simulink model "simulacion_validacion"  (R2022b)
settings: Solver=VariableStepAuto  StartTime=0.0  StopTime=50  RelTol=1e-3
values from neighbouring files (symbols this model uses):
  beta = gamma*2*I    (= 0.0001265)    [parametros.m]
  db = 4.2/100    (= 0.042)    [parametros.m]
  dc = 5/100    (= 0.05)    [parametros.m]
  dm = 13.1/100    (= 0.131)    [parametros.m]
  g = 9.81    [parametros.m]
  I = 1.1e-4    (= 0.00011)    [parametros.m]
  K = 0.001    [parametros.m]
  mb = 7.38/1000    (= 0.00738)    [parametros.m]
  mc = 2.07/1000    (= 0.00207)    [parametros.m]
  mm = (3.2+1.28)/1000    (= 0.00448)    [parametros.m]
settings Model: Creator=TAURET  LastModifiedBy=danie
settings DataIOCC: Refine=100
settings ModelReferenceCC: EnableRefExpFcnMdlSchedulingChecks=on

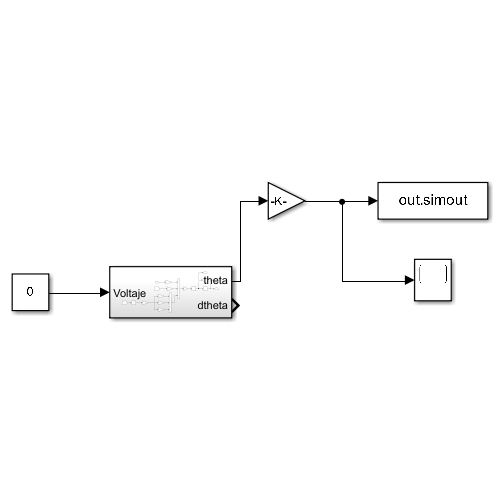
[thumbnail: Simulink's stored preview of the top-level diagram]
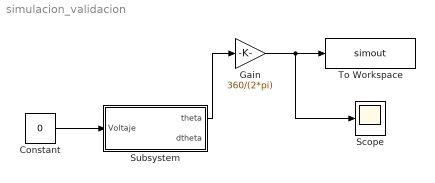
== system simulacion_validacion ==
  Constant : Constant  Value=0
  Gain : Gain  Gain=360/(2*pi)
  Scope : Scope
  Subsystem : Subsystem
  To Workspace : ToWorkspace  VariableName=simout  SaveFormat=Timeseries  SampleTime=-1
  wires:
  Subsystem/1(theta) -> Gain/1
  Gain/1 -> To Workspace/1, Scope/1
  Constant/1 -> Subsystem/1(Voltaje)

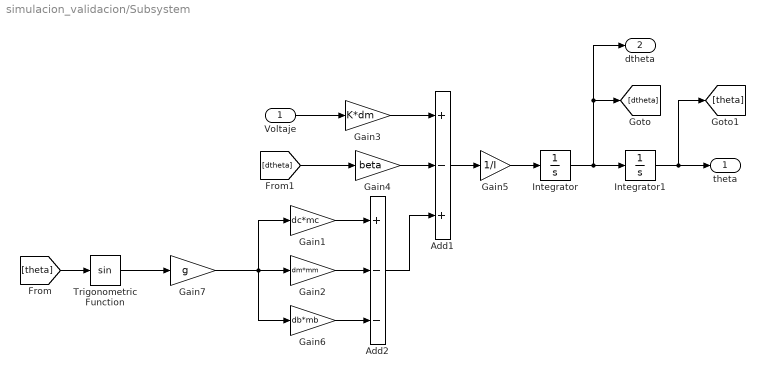
== system simulacion_validacion/Subsystem ==
  Voltaje : Inport
  Add1 : Sum  Inputs=+-+
  Add2 : Sum  Inputs=+--
  Gain1 : Gain  Gain=dc*mc
  Gain2 : Gain  Gain=dm*mm
  Gain3 : Gain  Gain=K*dm
  Gain4 : Gain  Gain=beta
  Gain5 : Gain  Gain=1/I
  Gain6 : Gain  Gain=db*mb
  Gain7 : Gain  Gain=g
  Integrator : Integrator
  Integrator1 : Integrator  InitialCondition=1.57
  Trigonometric Function : Trigonometry
  theta : Outport
  dtheta : Outport  Port=2
  wires:
  Gain4/1 -> Add1/2
  Gain5/1 -> Integrator/1
  Add1/1 -> Gain5/1
  [dtheta] -> Gain4/1
  [theta] -> Trigonometric Function/1
  Integrator/1 -> dtheta/1, [dtheta], Integrator1/1
  Integrator1/1 -> [theta], theta/1
  Voltaje/1 -> Gain3/1
  Gain1/1 -> Add2/1
  Gain2/1 -> Add2/2
  Gain6/1 -> Add2/3
  Add2/1 -> Add1/3
  Trigonometric Function/1 -> Gain7/1
  Gain3/1 -> Add1/1
  Gain7/1 -> Gain6/1, Gain2/1, Gain1/1
